simulink model "degrees_to_fahrenheit"  (R2015a)
settings: Solver=ode45  StartTime=0.0  StopTime=10.0  RelTol=1e-3
settings Model: Creator=Maina  LastModifiedBy=Maina

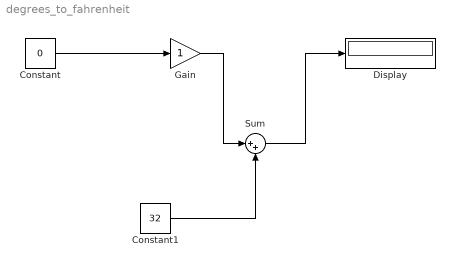
== system degrees_to_fahrenheit ==
  Constant : Constant  Value=0
  Constant1 : Constant  Value=32
  Display : Display
  Gain : Gain
  Sum : Sum  Inputs=|++
  wires:
  Constant1/1 -> Sum/2
  Gain/1 -> Sum/1
  Sum/1 -> Display/1
  Constant/1 -> Gain/1
